simulink model "Flip_Flop_Block"  (R2013b)
settings: Solver=ode45  StartTime=0.0  StopTime=10.0  RelTol=1e-3
libraries: tllib x1
settings Model: Creator=daltdoer  LastModifiedBy=daltdoer

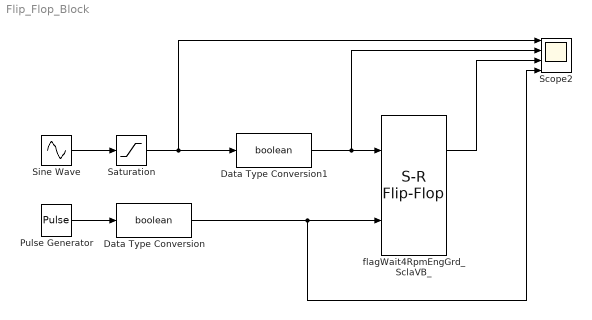
== system Flip_Flop_Block ==
  Data Type Conversion : DataTypeConversion  OutDataTypeStr=boolean  RndMeth=Round
  Data Type Conversion1 : DataTypeConversion  OutDataTypeStr=boolean  RndMeth=Nearest
  Pulse Generator : DiscretePulseGenerator  PulseType=Time based  Period=4  PulseWidth=20
  Saturation : Saturate  UpperLimit=1  LowerLimit=0
  Scope2 : Scope  NumInputPorts=4
      settings: YMin=-5~-5~-5~-5  YMax=5~5~5~5  SaveName=ScopeData2
  Sine Wave : Sin  SampleTime=0
  flagWait4RpmEngGrd_SclaVB_ : tllib/Extras/S-R Flip-Flop  Description=#user:hobruec#  initial_condition=0  data={'logdata',{'plotchannels',[]},'nlogdata',{'plotchannels',[]},'output',{'description',['Gradient der Motordrehzahl hat noch nicht Sollgradient erreicht']},'date',736211.52534859953}
  wires:
  flagWait4RpmEngGrd_SclaVB_/1 -> Scope2/3
  Sine Wave/1 -> Saturation/1
  Data Type Conversion/1 -> flagWait4RpmEngGrd_SclaVB_/2, Scope2/4
  Pulse Generator/1 -> Data Type Conversion/1
  Data Type Conversion1/1 -> Scope2/2, flagWait4RpmEngGrd_SclaVB_/1
  Saturation/1 -> Scope2/1, Data Type Conversion1/1
